simulink model "h175_model_stack_harness"  (R2023a)
settings: Solver=VariableStepAuto  StartTime=0.0  StopTime=4750  MaxStep=50  RelTol=1e-2
undefined symbols (not defined in the file): N2_T, sigbuilder_block
libraries: fl_lib x13, nesl_utility x11, SimscapeFluids_lib x2
(part 3 of 3)

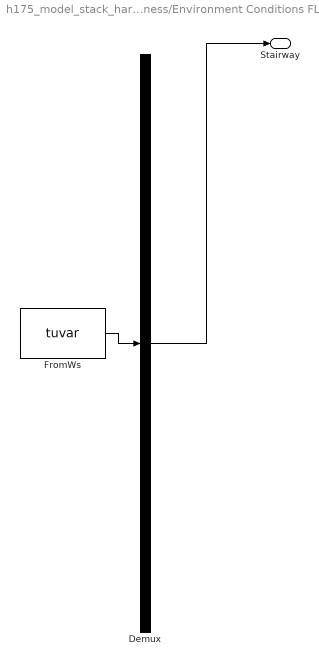
== system h175_model_stack_harness/Environment Conditions FL100 ==
  Demux : Demux  Tag=STV Demux  Outputs=1
      settings: DisplayOption=none
  FromWs : FromWorkspace  Tag=STV FromWs  VariableName=tuvar
      SigBuilderData=|
      | common.afterFinalStr = 'Extrapolate'
      | common.sampleTime = 0
      | dataSet.timeRange = [0 22226]
      | dataSet.name = 'Group 1'
      | sbobj.Groups.Name = 'Group 1'
      | sbobj.Groups.Signals.Name = 'Stairway'
      | sbobj.Groups.Signals.XData = [0 1 1.1 1.2 1.3 120 270 670 1450 7450 7510 21146 21826 22226]
      | sbobj.Groups.Signals.YData = [0 0 0 0 0 0 250 650 1100 1100 1000 1000 500 0]
      | sbobj.Groups.TimeRange = [0 22226]
  Stairway : Outport  Tag=STV Outport
  wires:
  Demux/1 -> Stairway/1
  FromWs/1 -> Demux/1

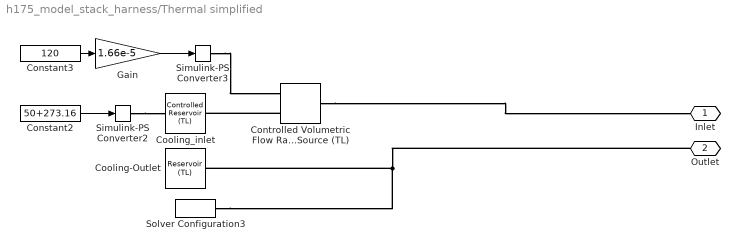
== system h175_model_stack_harness/Thermal simplified ==
  Constant2 : Constant  Value=50+273.16
  Constant3 : Constant  Value=120
  Controlled Volumetric Flow Rate Source (TL) : fl_lib/Thermal Liquid/Sources/Controlled Volumetric Flow Rate Source (TL)  power_spec=foundation.enum.power_spec.none  area=0.01 m^2
      settings: InternalSimscapePortConfiguration="{\"Bottom\":[],\"Left\":[{\"id\":\"A\",\"label\":\"A\",\"type\":\"foundation.thermal_liquid.thermal_liquid\"},{\"id\":\"V\",\"label\":\"V\",\"type\":\"input\"}],\"Right\":[{\"id\":\"B\",\"label\":\"B\",\"type\":\"foundation.thermal_liquid.thermal_liquid\"}],\"Top\":[]}"
  Cooling-Outlet : fl_lib/Thermal Liquid/Elements/Reservoir (TL)  pressure_spec=foundation.enum.pressure_spec.atmospheric  reservoir_pressure=0.101325 MPa  reservoir_temperature=293.15 K  area=0.01 m^2
  Cooling_inlet : fl_lib/Thermal Liquid/Elements/Controlled Reservoir (TL)  pressure_spec=foundation.enum.pressure_spec.specified  reservoir_pressure=3 bar  area=20 cm^2
      settings: InternalSimscapePortConfiguration="{\"Bottom\":[],\"Left\":[{\"id\":\"A\",\"label\":\"A\",\"type\":\"foundation.thermal_liquid.thermal_liquid\"}],\"Right\":[{\"id\":\"T_in\",\"label\":\"T\",\"type\":\"input\"}],\"Top\":[]}"
  Gain : Gain  Gain=1.66e-5
  Simulink-PS Converter2 : nesl_utility/Simulink-PS Converter  PhysicalDomain=network_engine_domain  SubClassName=ps_input  LeftPortType=input  RightPortType=output  PseudoPeriodic=off  Frequencies=[]  NoiseDistribution=none  NoiseParameters=[]  Unit=1  AffineConversion=off  FilteringAndDerivatives=provide  SimscapeFilterOrder=1  InputFilterTimeConstant=0.001  UdotUserProvided=0
  Simulink-PS Converter3 : nesl_utility/Simulink-PS Converter  PhysicalDomain=network_engine_domain  SubClassName=ps_input  LeftPortType=input  RightPortType=output  PseudoPeriodic=off  Frequencies=[]  NoiseDistribution=none  NoiseParameters=[]  Unit=1  AffineConversion=off  FilteringAndDerivatives=provide  SimscapeFilterOrder=1  InputFilterTimeConstant=0.001  UdotUserProvided=0
  Solver Configuration3 : nesl_utility/Solver Configuration  PhysicalDomain=network_engine_domain  SubClassName=solver  LeftPortType=input  RightPortType=generic  Tones=[]  Harmonics=[]  SimulateNoise=off  Profile=off  UseLocalSampling=off  EnableSwitchedLinearOptims=on  FrequencyDomain=off  UseCCode=off  RelTol=0.001  AbsTol=1e-06  MinStep=1e-09  ToWorkspace=off  RevertToSquareIcSolve=off  NumHomotopyIterations=100  PhasorMode=off  PhasorModeNumHarmonics=1  ConsistencySolver=NEWTON_XTOL_AFTER_FTOL  IndexReductionMethod=DerivativeReplacement  DoDC=off  ResidualTolerance=1e-09  ConsistencyTolSource=GLOBAL  ConsistencyAbsTol=0.001  ConsistencyRelTol=0.001  ConsistencyTolFactor=0.001  UseLocalSolver=on  LocalSolverChoice=NE_BACKWARD_EULER_ADVANCER  ResolveIndetEquations=on  FunctionEvalNumThread=1  LocalSolverSampleTime=0.001  DoFixedCost=on  MaxNonlinIter=3  MaxModeIter=2  ComputeImpulses=off  ImpulseIterations=2  LinearAlgebra=auto  LinearAlgebraNumThread=0  EquationFormulation=NE_TIME_EF  DelaysMemoryBudget=1024  AutomaticFiltering=off  FilteringTimeConstant=0.001  PartitionStorageMethod=AS_NEEDED  PartitionMemoryBudget=1024  PartitionMethod=ROBUST
  Inlet : PMIOPort  Side=Right
  Outlet : PMIOPort  Port=2  Side=Right
  wires:
  Constant2/1 -> Simulink-PS Converter2/1
  Gain/1 -> Simulink-PS Converter3/1
  Constant3/1 -> Gain/1
  connections:
  Controlled Volumetric Flow Rate Source (TL)/RConn1 -- Inlet/RConn1
  Simulink-PS Converter2/RConn1 -- Cooling_inlet/RConn1
  Controlled Volumetric Flow Rate Source (TL)/LConn1 -- Cooling_inlet/LConn1
  Simulink-PS Converter3/RConn1 -- Controlled Volumetric Flow Rate Source (TL)/LConn2
  Solver Configuration3/RConn1 -- Outlet/RConn1 -- Cooling-Outlet/LConn1
